simulink model "sampleModel1668_3"  (R2023a)
settings: Solver=VariableStepAuto  StartTime=0.0  StopTime=10.0  RelTol=1e-3
libraries: hdlsllib x7, simulink x1
settings Model: Creator=user1  LastModifiedBy=user1

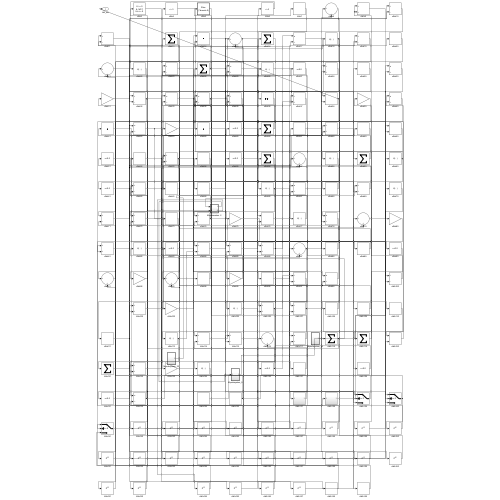
[thumbnail: Simulink's stored preview of the top-level diagram]
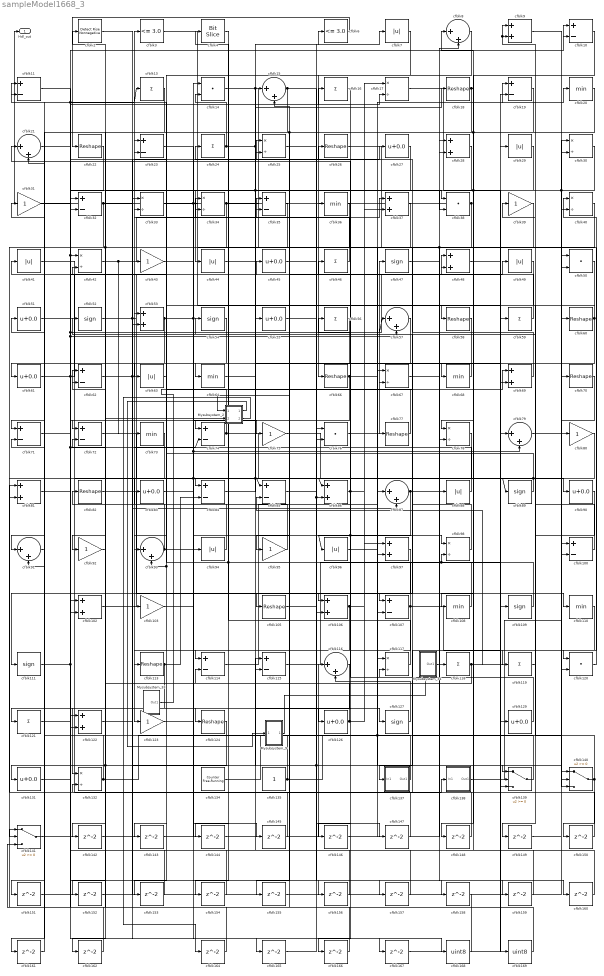
== system sampleModel1668_3 ==
  Mysubsystem_2 : Subsystem  TreatAsAtomicUnit=on  RTWFcnName=Mysubsystem_2
      settings: RTWFcnNameOpts=User specified  RTWFileNameOpts=Use function name
  Mysubsystem_33 : Subsystem  TreatAsAtomicUnit=on  RTWFcnName=Mysubsystem_33
      settings: RTWFcnNameOpts=User specified  RTWFileNameOpts=Use function name
  Mysubsystem_34 : Subsystem  TreatAsAtomicUnit=on  RTWFcnName=Mysubsystem_34
      settings: RTWFcnNameOpts=User specified  RTWFileNameOpts=Use function name
  Mysubsystem_9 : Subsystem  TreatAsAtomicUnit=on  RTWFcnName=Mysubsystem_9
      settings: RTWFcnNameOpts=User specified  RTWFileNameOpts=Use function name
  cfblk{10..11,19,23,32,35,62,71..72,74,84..85,100,107,114..115} (16 alike) : Sum  Inputs=+-  OutDataTypeStr=uint8
  cfblk{9,28,37,48,53,69,81,86,97,102,106,122} (12 alike) : Sum  OutDataTypeStr=uint8
  cfblk{31,39,43,75,80,92,95,103,123} (9 alike) : Gain  OutDataTypeStr=uint8
  cfblk{18,22,26,58,60,66,70,77,82,105,113,124} (12 alike) : Reshape
  cfblk{20,36,64,68,73,108,110} (7 alike) : MinMax  OutDataTypeStr=uint8
  cfblk{47,52,54,89,109,111,127} (7 alike) : Signum
  cfblk{8,15,21,57,79,87,91,93,116} (9 alike) : Sum  Inputs=|++  OutDataTypeStr=uint8
  cfblk{17,25,30,33..34,40,42,67,78,98,117,132} (12 alike) : Product  Inputs=*/  OutDataTypeStr=uint8  RndMeth=Zero  SaturateOnIntegerOverflow=on
  cfblk{13,16,24,46,56,59,118..119,121} (9 alike) : Sum  Inputs=+  OutDataTypeStr=uint8
  cfblk{14,38,50,76,120} (5 alike) : DotProduct  OutDataTypeStr=uint8
  cfblk{27,45,51,55,61,83,90,126,129,131} (10 alike) : Bias  Bias=0.0  SaturateOnIntegerOverflow=off
  cfblk134 : hdlsllib/Sources/Counter Free-Running  NumBits=16  tsamp=-1
  cfblk135 : Constant  OutDataTypeStr=uint8  SampleTime=-1
  cfblk137 : Subsystem
      settings: LibrarySourceBlock=|
      | hdlsllib/Ports &
      | Subsystems/Subsystem
  cfblk138 : Subsystem
      settings: LibrarySourceBlock=|
      | hdlsllib/Ports &
      | Subsystems/Subsystem
  cfblk139 : Switch  OutDataTypeStr=uint8  SaturateOnIntegerOverflow=off  InputSameDT=off
  cfblk140 : Switch  OutDataTypeStr=uint8  SaturateOnIntegerOverflow=off  InputSameDT=off
  cfblk141 : Switch  OutDataTypeStr=uint8  SaturateOnIntegerOverflow=off  InputSameDT=off
  cfblk{142..162,164..167} (25 alike) : Delay  SampleTime=1
  cfblk168 : DataTypeConversion  OutDataTypeStr=uint8  SaturateOnIntegerOverflow=off  RndMeth=Floor
  cfblk169 : DataTypeConversion  OutDataTypeStr=uint8  SaturateOnIntegerOverflow=off  RndMeth=Floor
  cfblk2 : hdlsllib/Logic and Bit Operations/Detect Rise Nonnegative  vinit=0  OutDataTypeStr=uint8
  cfblk{7,29,41,44,49,63,88,94,96} (9 alike) : Abs  OutDataTypeStr=uint8  SaturateOnIntegerOverflow=off
  cfblk3 : hdlsllib/Logic and Bit Operations/Compare To Constant  relop=<=  const=3.0  OutDataTypeStr=uint8
  cfblk4 : hdlsllib/Logic and Bit Operations/Bit Slice  lidx=7  ridx=0
  cfblk6 : hdlsllib/Logic and Bit Operations/Compare To Constant  relop=<=  const=3.0  OutDataTypeStr=uint8
  Hdl_out : Outport  OutDataTypeStr=uint8
  wires:
  cfblk119/1 -> cfblk54/1
  cfblk93/1 -> cfblk3/1, cfblk156/1
  cfblk51/1 -> cfblk138/1(In1)
  cfblk116/1 -> cfblk132/1
  cfblk74/1 -> cfblk90/1, cfblk43/1
  cfblk6/1 -> cfblk22/1
  cfblk135/1 -> cfblk50/1, cfblk77/1, cfblk72/2
  cfblk126/1 -> cfblk97/1, cfblk42/2
  cfblk26/1 -> cfblk120/1
  cfblk61/1 -> cfblk48/1, cfblk165/1
  cfblk73/1 -> cfblk123/1
  cfblk108/1 -> cfblk41/1, cfblk98/2
  cfblk30/1 -> cfblk68/1, cfblk144/1, cfblk50/2
  cfblk45/1 -> cfblk140/3, cfblk159/1
  cfblk39/1 -> cfblk107/1
  cfblk52/1 -> cfblk45/1, cfblk139/2
  cfblk19/1 -> cfblk71/1, cfblk108/1
  cfblk95/1 -> cfblk82/1
  cfblk11/1 -> cfblk38/1
  cfblk72/1 -> cfblk84/1
  cfblk82/1 -> cfblk110/1
  cfblk8/1 -> cfblk66/1
  cfblk13/1 -> cfblk131/1
  cfblk113/1 -> cfblk121/1, cfblk84/2
  cfblk102/1 -> cfblk46/1
  cfblk14/1 -> cfblk100/1, cfblk139/3
  cfblk76/1 -> cfblk47/1
  cfblk41/1 -> cfblk100/2
  cfblk92/1 -> cfblk62/1
  cfblk86/1 -> cfblk56/1, cfblk37/2
  cfblk3/1 -> cfblk109/1
  cfblk69/1 -> cfblk24/1
  cfblk120/1 -> cfblk40/1
  cfblk23/1 -> cfblk85/1, cfblk97/2
  cfblk89/1 -> cfblk86/1, cfblk23/2
  cfblk31/1 -> cfblk26/1
  cfblk59/1 -> cfblk25/1
  cfblk114/1 -> cfblk48/2
  cfblk22/1 -> cfblk32/2
  cfblk28/1 -> cfblk44/1
  cfblk53/1 -> cfblk17/2, cfblk98/1, cfblk92/1
  cfblk85/1 -> cfblk27/1
  cfblk58/1 -> cfblk96/1, cfblk126/1
  cfblk97/1 -> cfblk111/1
  cfblk106/1 -> cfblk113/1, cfblk17/1
  cfblk77/1 -> cfblk34/1
  cfblk100/1 -> cfblk39/1
  cfblk18/1 -> cfblk78/1, cfblk102/2
  cfblk20/1 -> Mysubsystem_2/1(In1), cfblk74/1
  cfblk44/1 -> cfblk69/2
  cfblk140/1 -> cfblk9/1, cfblk9/2, cfblk150/1
  cfblk98/1 -> cfblk52/1
  cfblk138/1(Out1) -> cfblk70/1
  cfblk78/1 -> cfblk141/2
  cfblk21/1 -> cfblk36/1
  cfblk25/1 -> cfblk38/2
  cfblk33/1 -> cfblk117/1, cfblk75/1
  cfblk63/1 -> cfblk93/2, cfblk153/1
  cfblk75/1 -> cfblk140/1
  cfblk91/1 -> cfblk31/1
  cfblk71/1 -> cfblk42/1, cfblk10/2
  cfblk81/1 -> cfblk13/1, cfblk10/1, cfblk57/2, cfblk74/2
  cfblk36/1 -> cfblk114/1
  cfblk46/1 -> cfblk33/2
  cfblk88/1 -> cfblk53/1
  cfblk117/1 -> cfblk34/2
  cfblk132/1 -> cfblk8/2, cfblk11/1
  cfblk29/1 -> cfblk115/2, cfblk142/1
  cfblk27/1 -> cfblk95/1
  cfblk129/1 -> cfblk21/1
  cfblk34/1 -> cfblk88/1, cfblk161/1
  cfblk62/1 -> cfblk29/1, cfblk25/2, cfblk158/1
  cfblk15/1 -> cfblk76/1, cfblk72/1
  cfblk55/1 -> cfblk7/1
  cfblk42/1 -> cfblk15/1, cfblk73/1
  cfblk115/1 -> cfblk79/1
  cfblk131/1 -> cfblk16/1, cfblk57/1
  cfblk96/1 -> cfblk19/1
  cfblk110/1 -> cfblk137/1(In1)
  cfblk109/1 -> cfblk4/1, cfblk11/2
  cfblk35/1 -> Mysubsystem_2/2(In2), cfblk91/1
  cfblk134/1 -> cfblk67/1
  cfblk7/1 -> cfblk103/1
  cfblk79/1 -> cfblk30/1
  cfblk103/1 -> cfblk79/2, cfblk37/1
  cfblk122/1 -> cfblk87/2
  cfblk107/1 -> cfblk35/1, cfblk129/1, cfblk166/1
  cfblk49/1 -> cfblk63/1
  cfblk68/1 -> cfblk64/1
  cfblk9/1 -> cfblk80/1
  cfblk17/1 -> cfblk59/1
  cfblk139/1 -> cfblk67/2
  cfblk57/1 -> cfblk105/1
  cfblk24/1 -> cfblk127/1, cfblk89/1, cfblk18/1, cfblk14/2
  cfblk43/1 -> cfblk94/1
  cfblk141/1 -> cfblk116/1
  cfblk127/1 -> cfblk116/2
  cfblk121/1 -> cfblk102/1
  cfblk84/1 -> cfblk55/1
  cfblk111/1 -> cfblk49/1, cfblk157/1
  cfblk118/1 -> cfblk60/1, cfblk114/2
  cfblk94/1 -> cfblk23/1
  cfblk60/1 -> cfblk58/1, cfblk93/1
  cfblk124/1 -> cfblk151/1, cfblk152/1
  cfblk40/1 -> cfblk86/2, cfblk106/2, cfblk78/2
  cfblk80/1 -> cfblk124/1
  cfblk70/1 -> cfblk140/2
  cfblk64/1 -> cfblk6/1
  cfblk87/1 -> cfblk106/1, cfblk20/1
  cfblk32/1 -> cfblk83/1, cfblk81/2
  cfblk47/1 -> cfblk28/1
  cfblk66/1 -> cfblk122/2, cfblk139/1
  cfblk137/1(Out1) -> cfblk21/2
  cfblk56/1 -> cfblk61/1
  cfblk50/1 -> cfblk119/1
  cfblk142/1 -> cfblk107/2
  cfblk54/1 -> cfblk143/1
  cfblk143/1 -> cfblk14/1
  cfblk144/1 -> cfblk28/2
  cfblk83/1 -> cfblk145/1
  cfblk145/1 -> cfblk33/1
  cfblk16/1 -> cfblk146/1
  cfblk146/1 -> cfblk87/1
  cfblk105/1 -> cfblk147/1
  cfblk147/1 -> cfblk71/2
  cfblk10/1 -> cfblk148/1
  cfblk148/1 -> cfblk117/2
  cfblk90/1 -> cfblk149/1
  cfblk149/1 -> cfblk120/2
  cfblk150/1 -> cfblk81/1
  cfblk151/1 -> cfblk30/2
  cfblk152/1 -> cfblk53/2
  cfblk153/1 -> cfblk62/2
  cfblk4/1 -> cfblk154/1
  cfblk154/1 -> cfblk32/1
  cfblk38/1 -> cfblk155/1, Hdl_out/1
  cfblk155/1 -> cfblk40/2
  cfblk156/1 -> cfblk35/2
  cfblk157/1 -> cfblk115/1
  cfblk158/1 -> cfblk141/3
  cfblk159/1 -> cfblk8/1
  cfblk67/1 -> cfblk160/1
  cfblk160/1 -> cfblk132/2
  cfblk161/1 -> cfblk91/2
  cfblk37/1 -> cfblk162/1
  cfblk162/1 -> cfblk122/1
  cfblk164/1 -> cfblk141/1
  cfblk165/1 -> cfblk76/2
  cfblk166/1 -> cfblk15/2
  cfblk123/1 -> cfblk167/1
  cfblk167/1 -> cfblk19/2
  cfblk2/1 -> cfblk168/1
  cfblk168/1 -> cfblk51/1
  cfblk48/1 -> cfblk169/1
  cfblk169/1 -> cfblk2/1
  Mysubsystem_2/2(Out2) -> cfblk164/1
  Mysubsystem_2/1(Out1) -> Mysubsystem_9/1(In1)
  Mysubsystem_9/1(Out1) -> cfblk118/1
  Mysubsystem_33/1(Out1) -> cfblk69/1
  Mysubsystem_34/1(Out1) -> cfblk85/2

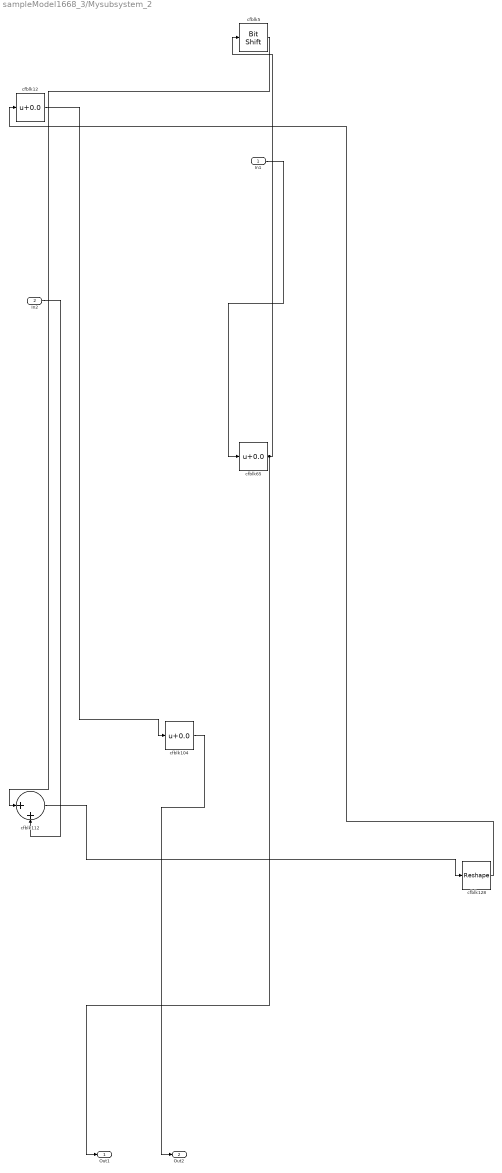
== system sampleModel1668_3/Mysubsystem_2 ==
  In1 : Inport
  In2 : Inport  Port=2
  cfblk104 : Bias  Bias=0.0  SaturateOnIntegerOverflow=off
  cfblk112 : Sum  Inputs=|++
  cfblk12 : Bias  Bias=0.0  SaturateOnIntegerOverflow=off
  cfblk128 : Reshape
  cfblk5 : hdlsllib/Logic and Bit Operations/Bit Shift  mode=Shift Left Logical  N=0
  cfblk65 : Bias  Bias=0.0  SaturateOnIntegerOverflow=off
  Out1 : Outport
  Out2 : Outport  Port=2
  wires:
  cfblk128/1 -> cfblk12/1
  cfblk12/1 -> cfblk104/1
  cfblk112/1 -> cfblk128/1
  cfblk5/1 -> cfblk112/1
  cfblk104/1 -> Out2/1
  cfblk65/1 -> Out1/1, cfblk5/1
  In1/1 -> cfblk65/1
  In2/1 -> cfblk112/2

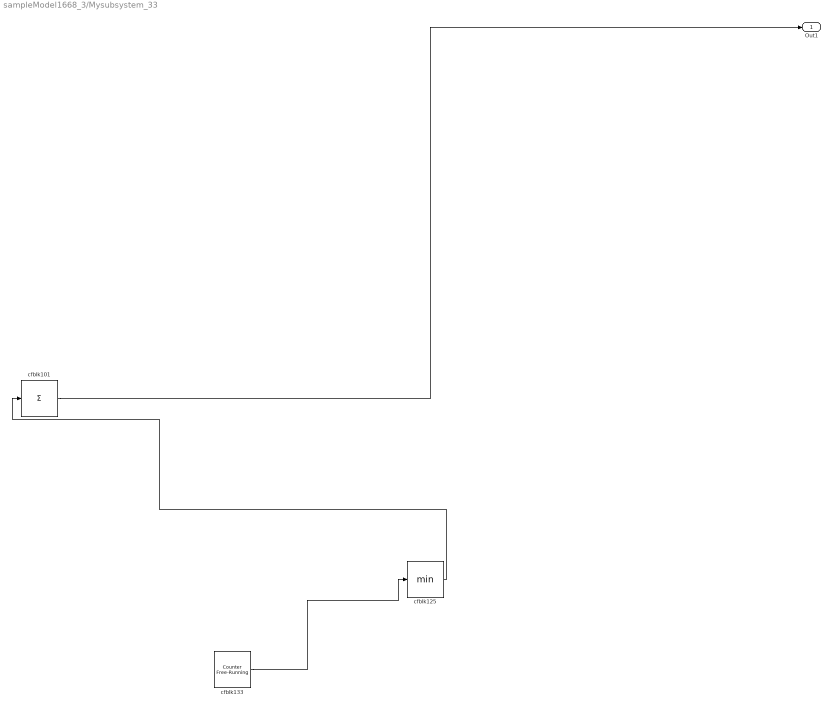
== system sampleModel1668_3/Mysubsystem_33 ==
  cfblk101 : Sum  Inputs=+
  cfblk125 : MinMax
  cfblk133 : hdlsllib/Sources/Counter Free-Running  NumBits=16  tsamp=-1
  Out1 : Outport
  wires:
  cfblk125/1 -> cfblk101/1
  cfblk133/1 -> cfblk125/1
  cfblk101/1 -> Out1/1

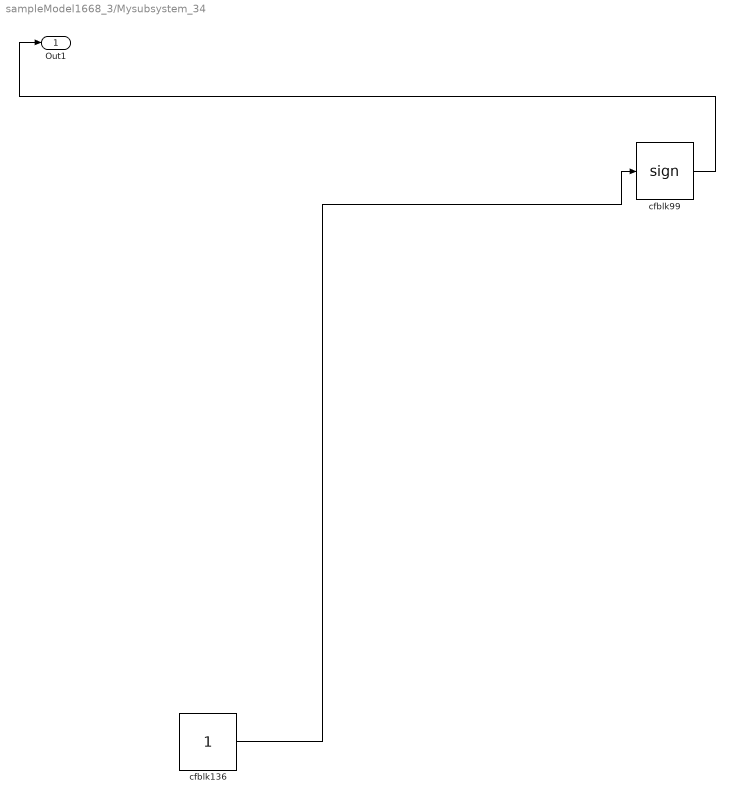
== system sampleModel1668_3/Mysubsystem_34 ==
  cfblk136 : Constant  SampleTime=-1
  cfblk99 : Signum
  Out1 : Outport
  wires:
  cfblk136/1 -> cfblk99/1
  cfblk99/1 -> Out1/1

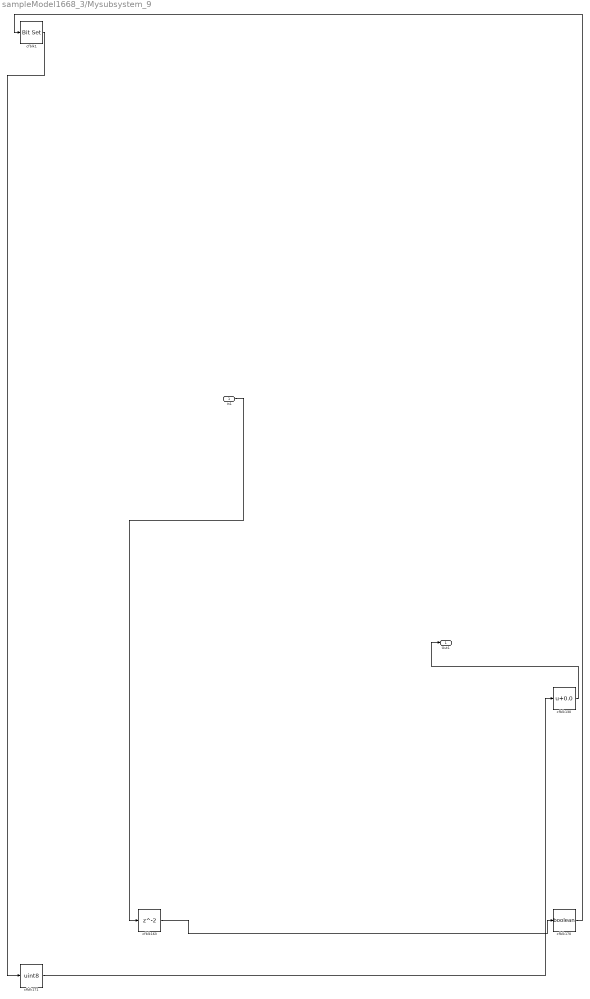
== system sampleModel1668_3/Mysubsystem_9 ==
  In1 : Inport
  cfblk1 : simulink/Logic and Bit Operations/Bit Set  iBit=0
      settings: LibrarySourceBlock=|
      | hdlsllib/Logic and Bit
      | Operations/Bit Set
  cfblk130 : Bias  Bias=0.0  SaturateOnIntegerOverflow=off
  cfblk163 : Delay  SampleTime=1
  cfblk170 : DataTypeConversion  OutDataTypeStr=boolean  SaturateOnIntegerOverflow=off  RndMeth=Floor
  cfblk171 : DataTypeConversion  OutDataTypeStr=uint8  SaturateOnIntegerOverflow=off  RndMeth=Floor
  Out1 : Outport
  wires:
  cfblk163/1 -> cfblk170/1
  cfblk171/1 -> cfblk130/1
  cfblk1/1 -> cfblk171/1
  cfblk130/1 -> Out1/1
  In1/1 -> cfblk163/1
  cfblk170/1 -> cfblk1/1

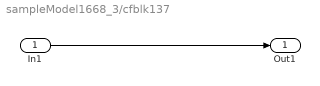
== system sampleModel1668_3/cfblk137 ==
  In1 : Inport
  Out1 : Outport
  wires:
  In1/1 -> Out1/1

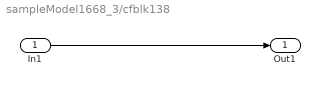
== system sampleModel1668_3/cfblk138 ==
  In1 : Inport
  Out1 : Outport
  wires:
  In1/1 -> Out1/1
